simulink model "VACModel"  (Simulink 8.3)
settings: Solver=ode1  SolverMode=MultiTasking  StartTime=0.0  StopTime=24  FixedStep=Ts_base  MaxStep=Ts_base  MinStep=1e-6  RelTol=1e-6
PreLoadFcn:
  | initModel
StopFcn:
  | overview
undefined symbols (not defined in the file): automatic, controller_sampling_frequency, Fixed, gcr, MVs, PI, signal, transmitter_deadtime, transmitter_sampling_frequency, Ts_save, y_ss
libraries: VAlib x96
(part 12 of 18)

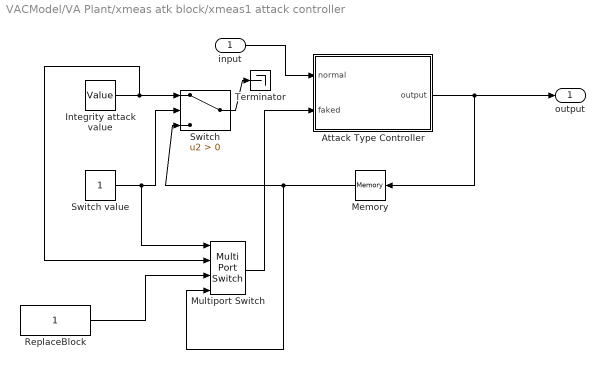
== system VACModel/VA Plant/xmeas atk block/xmeas1 attack controller ==
  input : Inport
  Attack Type Controller : Subsystem  Variant=on  OverrideUsingVariant=normal_forward_controller  mask{atkMode=No attack, start=0, duration=duration}
      mask prompts: atkMode "Attack Mode:"
      mask TypeOptions atkMode: No attack | Step attack | Interval attack | Periodical attack
      mask Callback atkMode:
      | switch get_param(gcb,'atkMode');
      |     case 'Step attack'
      |         set_param(gcb, 'OverrideUsingVariant', 'step_forward_controller');
      |     case 'Interval attack'
      |         set_param(gcb, 'OverrideUsingVariant', 'interval_forward_controller');
      |     case 'Periodical attack'
      |         set_param(gcb, 'OverrideUsingVariant', 'periodical_forward_controller');
      |     otherwise
      |         set_param(gcb, 'OverrideUsingVariant', 'normal_forward_controller');
      | end
      mask Display: eval(get_param([gcb '/' strrep(get_param(gcb, 'ActiveVariant'), '_', ' ')], 'MaskDisplay'));
  Integrity attack value : Constant  Value=Value
  Memory : Memory
  Multiport Switch : MultiPortSwitch
  ReplaceBlock : Constant
  Switch : Switch  Criteria=u2 > Threshold
  Switch value : Constant
  Terminator : Terminator
  output : Outport
  wires:
  ReplaceBlock/1 -> Multiport Switch/3
  Switch/1 -> Terminator/1
  Multiport Switch/1 -> Attack Type Controller/2(faked)
  Memory/1 -> Switch/3, Multiport Switch/4
  input/1 -> Attack Type Controller/1(normal)
  Switch value/1 -> Switch/2, Multiport Switch/1
  Attack Type Controller/1(output) -> output/1, Memory/1
  Integrity attack value/1 -> Switch/1, Multiport Switch/2

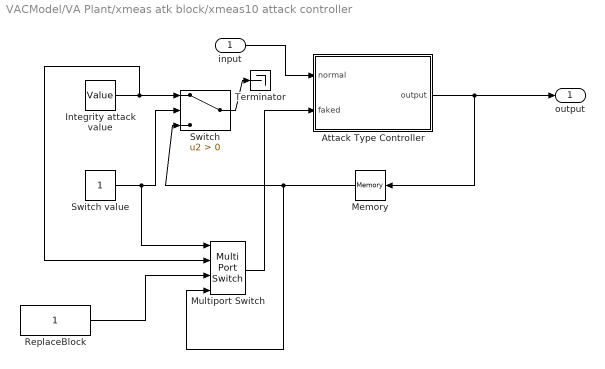
== system VACModel/VA Plant/xmeas atk block/xmeas10 attack controller ==
  input : Inport
  Attack Type Controller : Subsystem  Variant=on  OverrideUsingVariant=normal_forward_controller  mask{atkMode=No attack, start=0, duration=duration}
      mask prompts: atkMode "Attack Mode:"
      mask TypeOptions atkMode: No attack | Step attack | Interval attack | Periodical attack
      mask Callback atkMode:
      | switch get_param(gcb,'atkMode');
      |     case 'Step attack'
      |         set_param(gcb, 'OverrideUsingVariant', 'step_forward_controller');
      |     case 'Interval attack'
      |         set_param(gcb, 'OverrideUsingVariant', 'interval_forward_controller');
      |     case 'Periodical attack'
      |         set_param(gcb, 'OverrideUsingVariant', 'periodical_forward_controller');
      |     otherwise
      |         set_param(gcb, 'OverrideUsingVariant', 'normal_forward_controller');
      | end
      mask Display: eval(get_param([gcb '/' strrep(get_param(gcb, 'ActiveVariant'), '_', ' ')], 'MaskDisplay'));
  Integrity attack value : Constant  Value=Value
  Memory : Memory
  Multiport Switch : MultiPortSwitch
  ReplaceBlock : Constant
  Switch : Switch  Criteria=u2 > Threshold
  Switch value : Constant
  Terminator : Terminator
  output : Outport
  wires:
  ReplaceBlock/1 -> Multiport Switch/3
  Switch/1 -> Terminator/1
  Multiport Switch/1 -> Attack Type Controller/2(faked)
  Memory/1 -> Switch/3, Multiport Switch/4
  input/1 -> Attack Type Controller/1(normal)
  Switch value/1 -> Switch/2, Multiport Switch/1
  Attack Type Controller/1(output) -> output/1, Memory/1
  Integrity attack value/1 -> Switch/1, Multiport Switch/2

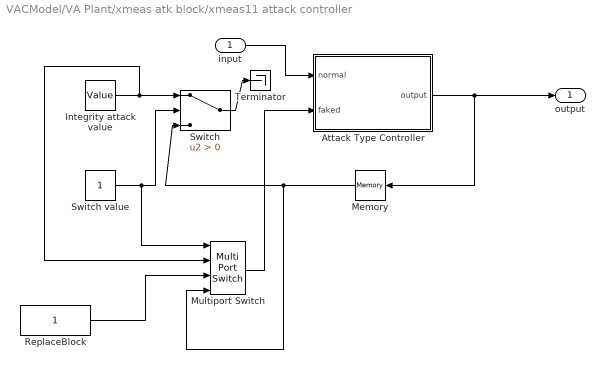
== system VACModel/VA Plant/xmeas atk block/xmeas11 attack controller ==
  input : Inport
  Attack Type Controller : Subsystem  Variant=on  OverrideUsingVariant=normal_forward_controller  mask{atkMode=No attack, start=0, duration=duration}
      mask prompts: atkMode "Attack Mode:"
      mask TypeOptions atkMode: No attack | Step attack | Interval attack | Periodical attack
      mask Callback atkMode:
      | switch get_param(gcb,'atkMode');
      |     case 'Step attack'
      |         set_param(gcb, 'OverrideUsingVariant', 'step_forward_controller');
      |     case 'Interval attack'
      |         set_param(gcb, 'OverrideUsingVariant', 'interval_forward_controller');
      |     case 'Periodical attack'
      |         set_param(gcb, 'OverrideUsingVariant', 'periodical_forward_controller');
      |     otherwise
      |         set_param(gcb, 'OverrideUsingVariant', 'normal_forward_controller');
      | end
      mask Display: eval(get_param([gcb '/' strrep(get_param(gcb, 'ActiveVariant'), '_', ' ')], 'MaskDisplay'));
  Integrity attack value : Constant  Value=Value
  Memory : Memory
  Multiport Switch : MultiPortSwitch
  ReplaceBlock : Constant
  Switch : Switch  Criteria=u2 > Threshold
  Switch value : Constant
  Terminator : Terminator
  output : Outport
  wires:
  ReplaceBlock/1 -> Multiport Switch/3
  Switch/1 -> Terminator/1
  Multiport Switch/1 -> Attack Type Controller/2(faked)
  Memory/1 -> Switch/3, Multiport Switch/4
  input/1 -> Attack Type Controller/1(normal)
  Switch value/1 -> Switch/2, Multiport Switch/1
  Attack Type Controller/1(output) -> output/1, Memory/1
  Integrity attack value/1 -> Switch/1, Multiport Switch/2

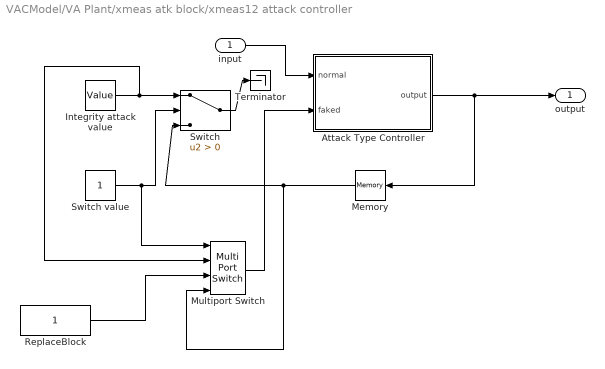
== system VACModel/VA Plant/xmeas atk block/xmeas12 attack controller ==
  input : Inport
  Attack Type Controller : Subsystem  Variant=on  OverrideUsingVariant=normal_forward_controller  mask{atkMode=No attack, start=0, duration=duration}
      mask prompts: atkMode "Attack Mode:"
      mask TypeOptions atkMode: No attack | Step attack | Interval attack | Periodical attack
      mask Callback atkMode:
      | switch get_param(gcb,'atkMode');
      |     case 'Step attack'
      |         set_param(gcb, 'OverrideUsingVariant', 'step_forward_controller');
      |     case 'Interval attack'
      |         set_param(gcb, 'OverrideUsingVariant', 'interval_forward_controller');
      |     case 'Periodical attack'
      |         set_param(gcb, 'OverrideUsingVariant', 'periodical_forward_controller');
      |     otherwise
      |         set_param(gcb, 'OverrideUsingVariant', 'normal_forward_controller');
      | end
      mask Display: eval(get_param([gcb '/' strrep(get_param(gcb, 'ActiveVariant'), '_', ' ')], 'MaskDisplay'));
  Integrity attack value : Constant  Value=Value
  Memory : Memory
  Multiport Switch : MultiPortSwitch
  ReplaceBlock : Constant
  Switch : Switch  Criteria=u2 > Threshold
  Switch value : Constant
  Terminator : Terminator
  output : Outport
  wires:
  ReplaceBlock/1 -> Multiport Switch/3
  Switch/1 -> Terminator/1
  Multiport Switch/1 -> Attack Type Controller/2(faked)
  Memory/1 -> Switch/3, Multiport Switch/4
  input/1 -> Attack Type Controller/1(normal)
  Switch value/1 -> Switch/2, Multiport Switch/1
  Attack Type Controller/1(output) -> output/1, Memory/1
  Integrity attack value/1 -> Switch/1, Multiport Switch/2

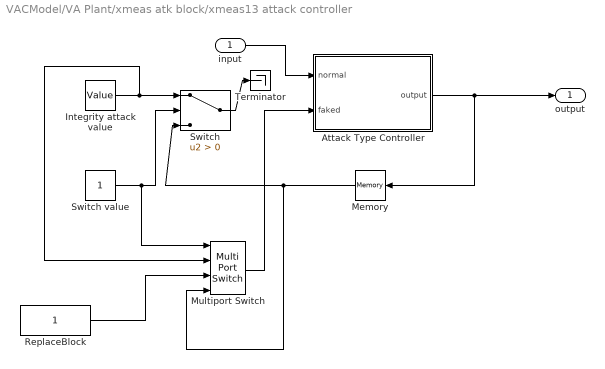
== system VACModel/VA Plant/xmeas atk block/xmeas13 attack controller ==
  input : Inport
  Attack Type Controller : Subsystem  Variant=on  OverrideUsingVariant=normal_forward_controller  mask{atkMode=No attack, start=0, duration=duration}
      mask prompts: atkMode "Attack Mode:"
      mask TypeOptions atkMode: No attack | Step attack | Interval attack | Periodical attack
      mask Callback atkMode:
      | switch get_param(gcb,'atkMode');
      |     case 'Step attack'
      |         set_param(gcb, 'OverrideUsingVariant', 'step_forward_controller');
      |     case 'Interval attack'
      |         set_param(gcb, 'OverrideUsingVariant', 'interval_forward_controller');
      |     case 'Periodical attack'
      |         set_param(gcb, 'OverrideUsingVariant', 'periodical_forward_controller');
      |     otherwise
      |         set_param(gcb, 'OverrideUsingVariant', 'normal_forward_controller');
      | end
      mask Display: eval(get_param([gcb '/' strrep(get_param(gcb, 'ActiveVariant'), '_', ' ')], 'MaskDisplay'));
  Integrity attack value : Constant  Value=Value
  Memory : Memory
  Multiport Switch : MultiPortSwitch
  ReplaceBlock : Constant
  Switch : Switch  Criteria=u2 > Threshold
  Switch value : Constant
  Terminator : Terminator
  output : Outport
  wires:
  ReplaceBlock/1 -> Multiport Switch/3
  Switch/1 -> Terminator/1
  Multiport Switch/1 -> Attack Type Controller/2(faked)
  Memory/1 -> Switch/3, Multiport Switch/4
  input/1 -> Attack Type Controller/1(normal)
  Switch value/1 -> Switch/2, Multiport Switch/1
  Attack Type Controller/1(output) -> output/1, Memory/1
  Integrity attack value/1 -> Switch/1, Multiport Switch/2

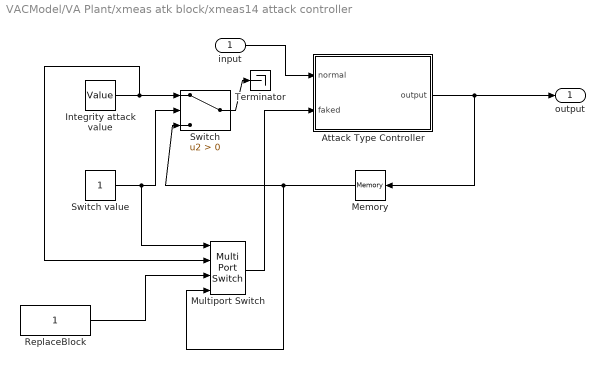
== system VACModel/VA Plant/xmeas atk block/xmeas14 attack controller ==
  input : Inport
  Attack Type Controller : Subsystem  Variant=on  OverrideUsingVariant=normal_forward_controller  mask{atkMode=No attack, start=0, duration=duration}
      mask prompts: atkMode "Attack Mode:"
      mask TypeOptions atkMode: No attack | Step attack | Interval attack | Periodical attack
      mask Callback atkMode:
      | switch get_param(gcb,'atkMode');
      |     case 'Step attack'
      |         set_param(gcb, 'OverrideUsingVariant', 'step_forward_controller');
      |     case 'Interval attack'
      |         set_param(gcb, 'OverrideUsingVariant', 'interval_forward_controller');
      |     case 'Periodical attack'
      |         set_param(gcb, 'OverrideUsingVariant', 'periodical_forward_controller');
      |     otherwise
      |         set_param(gcb, 'OverrideUsingVariant', 'normal_forward_controller');
      | end
      mask Display: eval(get_param([gcb '/' strrep(get_param(gcb, 'ActiveVariant'), '_', ' ')], 'MaskDisplay'));
  Integrity attack value : Constant  Value=Value
  Memory : Memory
  Multiport Switch : MultiPortSwitch
  ReplaceBlock : Constant
  Switch : Switch  Criteria=u2 > Threshold
  Switch value : Constant
  Terminator : Terminator
  output : Outport
  wires:
  ReplaceBlock/1 -> Multiport Switch/3
  Switch/1 -> Terminator/1
  Multiport Switch/1 -> Attack Type Controller/2(faked)
  Memory/1 -> Switch/3, Multiport Switch/4
  input/1 -> Attack Type Controller/1(normal)
  Switch value/1 -> Switch/2, Multiport Switch/1
  Attack Type Controller/1(output) -> output/1, Memory/1
  Integrity attack value/1 -> Switch/1, Multiport Switch/2

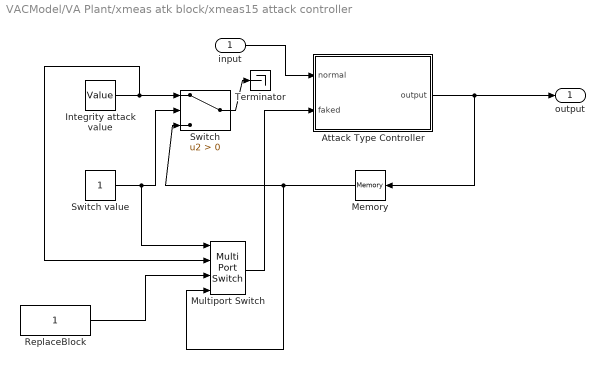
== system VACModel/VA Plant/xmeas atk block/xmeas15 attack controller ==
  input : Inport
  Attack Type Controller : Subsystem  Variant=on  OverrideUsingVariant=normal_forward_controller  mask{atkMode=No attack, start=0, duration=duration}
      mask prompts: atkMode "Attack Mode:"
      mask TypeOptions atkMode: No attack | Step attack | Interval attack | Periodical attack
      mask Callback atkMode:
      | switch get_param(gcb,'atkMode');
      |     case 'Step attack'
      |         set_param(gcb, 'OverrideUsingVariant', 'step_forward_controller');
      |     case 'Interval attack'
      |         set_param(gcb, 'OverrideUsingVariant', 'interval_forward_controller');
      |     case 'Periodical attack'
      |         set_param(gcb, 'OverrideUsingVariant', 'periodical_forward_controller');
      |     otherwise
      |         set_param(gcb, 'OverrideUsingVariant', 'normal_forward_controller');
      | end
      mask Display: eval(get_param([gcb '/' strrep(get_param(gcb, 'ActiveVariant'), '_', ' ')], 'MaskDisplay'));
  Integrity attack value : Constant  Value=Value
  Memory : Memory
  Multiport Switch : MultiPortSwitch
  ReplaceBlock : Constant
  Switch : Switch  Criteria=u2 > Threshold
  Switch value : Constant
  Terminator : Terminator
  output : Outport
  wires:
  ReplaceBlock/1 -> Multiport Switch/3
  Switch/1 -> Terminator/1
  Multiport Switch/1 -> Attack Type Controller/2(faked)
  Memory/1 -> Switch/3, Multiport Switch/4
  input/1 -> Attack Type Controller/1(normal)
  Switch value/1 -> Switch/2, Multiport Switch/1
  Attack Type Controller/1(output) -> output/1, Memory/1
  Integrity attack value/1 -> Switch/1, Multiport Switch/2

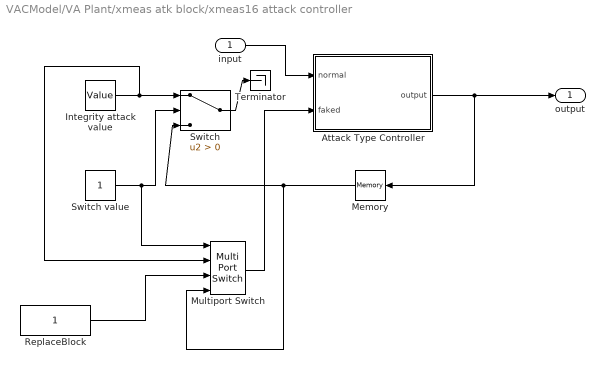
== system VACModel/VA Plant/xmeas atk block/xmeas16 attack controller ==
  input : Inport
  Attack Type Controller : Subsystem  Variant=on  OverrideUsingVariant=normal_forward_controller  mask{atkMode=No attack, start=0, duration=duration}
      mask prompts: atkMode "Attack Mode:"
      mask TypeOptions atkMode: No attack | Step attack | Interval attack | Periodical attack
      mask Callback atkMode:
      | switch get_param(gcb,'atkMode');
      |     case 'Step attack'
      |         set_param(gcb, 'OverrideUsingVariant', 'step_forward_controller');
      |     case 'Interval attack'
      |         set_param(gcb, 'OverrideUsingVariant', 'interval_forward_controller');
      |     case 'Periodical attack'
      |         set_param(gcb, 'OverrideUsingVariant', 'periodical_forward_controller');
      |     otherwise
      |         set_param(gcb, 'OverrideUsingVariant', 'normal_forward_controller');
      | end
      mask Display: eval(get_param([gcb '/' strrep(get_param(gcb, 'ActiveVariant'), '_', ' ')], 'MaskDisplay'));
  Integrity attack value : Constant  Value=Value
  Memory : Memory
  Multiport Switch : MultiPortSwitch
  ReplaceBlock : Constant
  Switch : Switch  Criteria=u2 > Threshold
  Switch value : Constant
  Terminator : Terminator
  output : Outport
  wires:
  ReplaceBlock/1 -> Multiport Switch/3
  Switch/1 -> Terminator/1
  Multiport Switch/1 -> Attack Type Controller/2(faked)
  Memory/1 -> Switch/3, Multiport Switch/4
  input/1 -> Attack Type Controller/1(normal)
  Switch value/1 -> Switch/2, Multiport Switch/1
  Attack Type Controller/1(output) -> output/1, Memory/1
  Integrity attack value/1 -> Switch/1, Multiport Switch/2

== system VACModel/VA Plant/xmeas atk block/xmeas17 attack controller ==
  input : Inport
  Attack Type Controller : Subsystem  Variant=on  OverrideUsingVariant=normal_forward_controller  mask{atkMode=No attack, start=0, duration=duration}
      mask prompts: atkMode "Attack Mode:"
      mask TypeOptions atkMode: No attack | Step attack | Interval attack | Periodical attack
      mask Callback atkMode:
      | switch get_param(gcb,'atkMode');
      |     case 'Step attack'
      |         set_param(gcb, 'OverrideUsingVariant', 'step_forward_controller');
      |     case 'Interval attack'
      |         set_param(gcb, 'OverrideUsingVariant', 'interval_forward_controller');
      |     case 'Periodical attack'
      |         set_param(gcb, 'OverrideUsingVariant', 'periodical_forward_controller');
      |     otherwise
      |         set_param(gcb, 'OverrideUsingVariant', 'normal_forward_controller');
      | end
      mask Display: eval(get_param([gcb '/' strrep(get_param(gcb, 'ActiveVariant'), '_', ' ')], 'MaskDisplay'));
  Integrity attack value : Constant  Value=Value
  Memory : Memory
  Multiport Switch : MultiPortSwitch
  ReplaceBlock : Constant
  Switch : Switch  Criteria=u2 > Threshold
  Switch value : Constant
  Terminator : Terminator
  output : Outport
  wires:
  ReplaceBlock/1 -> Multiport Switch/3
  Switch/1 -> Terminator/1
  Multiport Switch/1 -> Attack Type Controller/2(faked)
  Memory/1 -> Switch/3, Multiport Switch/4
  input/1 -> Attack Type Controller/1(normal)
  Switch value/1 -> Switch/2, Multiport Switch/1
  Attack Type Controller/1(output) -> output/1, Memory/1
  Integrity attack value/1 -> Switch/1, Multiport Switch/2

== system VACModel/VA Plant/xmeas atk block/xmeas18 attack controller ==
  input : Inport
  Attack Type Controller : Subsystem  Variant=on  OverrideUsingVariant=normal_forward_controller  mask{atkMode=No attack, start=0, duration=duration}
      mask prompts: atkMode "Attack Mode:"
      mask TypeOptions atkMode: No attack | Step attack | Interval attack | Periodical attack
      mask Callback atkMode:
      | switch get_param(gcb,'atkMode');
      |     case 'Step attack'
      |         set_param(gcb, 'OverrideUsingVariant', 'step_forward_controller');
      |     case 'Interval attack'
      |         set_param(gcb, 'OverrideUsingVariant', 'interval_forward_controller');
      |     case 'Periodical attack'
      |         set_param(gcb, 'OverrideUsingVariant', 'periodical_forward_controller');
      |     otherwise
      |         set_param(gcb, 'OverrideUsingVariant', 'normal_forward_controller');
      | end
      mask Display: eval(get_param([gcb '/' strrep(get_param(gcb, 'ActiveVariant'), '_', ' ')], 'MaskDisplay'));
  Integrity attack value : Constant  Value=Value
  Memory : Memory
  Multiport Switch : MultiPortSwitch
  ReplaceBlock : Constant
  Switch : Switch  Criteria=u2 > Threshold
  Switch value : Constant
  Terminator : Terminator
  output : Outport
  wires:
  ReplaceBlock/1 -> Multiport Switch/3
  Switch/1 -> Terminator/1
  Multiport Switch/1 -> Attack Type Controller/2(faked)
  Memory/1 -> Switch/3, Multiport Switch/4
  input/1 -> Attack Type Controller/1(normal)
  Switch value/1 -> Switch/2, Multiport Switch/1
  Attack Type Controller/1(output) -> output/1, Memory/1
  Integrity attack value/1 -> Switch/1, Multiport Switch/2

== system VACModel/VA Plant/xmeas atk block/xmeas19 attack controller ==
  input : Inport
  Attack Type Controller : Subsystem  Variant=on  OverrideUsingVariant=normal_forward_controller  mask{atkMode=No attack, start=0, duration=duration}
      mask prompts: atkMode "Attack Mode:"
      mask TypeOptions atkMode: No attack | Step attack | Interval attack | Periodical attack
      mask Callback atkMode:
      | switch get_param(gcb,'atkMode');
      |     case 'Step attack'
      |         set_param(gcb, 'OverrideUsingVariant', 'step_forward_controller');
      |     case 'Interval attack'
      |         set_param(gcb, 'OverrideUsingVariant', 'interval_forward_controller');
      |     case 'Periodical attack'
      |         set_param(gcb, 'OverrideUsingVariant', 'periodical_forward_controller');
      |     otherwise
      |         set_param(gcb, 'OverrideUsingVariant', 'normal_forward_controller');
      | end
      mask Display: eval(get_param([gcb '/' strrep(get_param(gcb, 'ActiveVariant'), '_', ' ')], 'MaskDisplay'));
  Integrity attack value : Constant  Value=Value
  Memory : Memory
  Multiport Switch : MultiPortSwitch
  ReplaceBlock : Constant
  Switch : Switch  Criteria=u2 > Threshold
  Switch value : Constant
  Terminator : Terminator
  output : Outport
  wires:
  ReplaceBlock/1 -> Multiport Switch/3
  Switch/1 -> Terminator/1
  Multiport Switch/1 -> Attack Type Controller/2(faked)
  Memory/1 -> Switch/3, Multiport Switch/4
  input/1 -> Attack Type Controller/1(normal)
  Switch value/1 -> Switch/2, Multiport Switch/1
  Attack Type Controller/1(output) -> output/1, Memory/1
  Integrity attack value/1 -> Switch/1, Multiport Switch/2

== system VACModel/VA Plant/xmeas atk block/xmeas2 attack controller ==
  input : Inport
  Attack Type Controller : Subsystem  Variant=on  OverrideUsingVariant=normal_forward_controller  mask{atkMode=No attack, start=0, duration=duration}
      mask prompts: atkMode "Attack Mode:"
      mask TypeOptions atkMode: No attack | Step attack | Interval attack | Periodical attack
      mask Callback atkMode:
      | switch get_param(gcb,'atkMode');
      |     case 'Step attack'
      |         set_param(gcb, 'OverrideUsingVariant', 'step_forward_controller');
      |     case 'Interval attack'
      |         set_param(gcb, 'OverrideUsingVariant', 'interval_forward_controller');
      |     case 'Periodical attack'
      |         set_param(gcb, 'OverrideUsingVariant', 'periodical_forward_controller');
      |     otherwise
      |         set_param(gcb, 'OverrideUsingVariant', 'normal_forward_controller');
      | end
      mask Display: eval(get_param([gcb '/' strrep(get_param(gcb, 'ActiveVariant'), '_', ' ')], 'MaskDisplay'));
  Integrity attack value : Constant  Value=Value
  Memory : Memory
  Multiport Switch : MultiPortSwitch
  ReplaceBlock : Constant
  Switch : Switch  Criteria=u2 > Threshold
  Switch value : Constant
  Terminator : Terminator
  output : Outport
  wires:
  ReplaceBlock/1 -> Multiport Switch/3
  Switch/1 -> Terminator/1
  Multiport Switch/1 -> Attack Type Controller/2(faked)
  Memory/1 -> Switch/3, Multiport Switch/4
  input/1 -> Attack Type Controller/1(normal)
  Switch value/1 -> Switch/2, Multiport Switch/1
  Attack Type Controller/1(output) -> output/1, Memory/1
  Integrity attack value/1 -> Switch/1, Multiport Switch/2

== system VACModel/VA Plant/xmeas atk block/xmeas20 attack controller ==
  input : Inport
  Attack Type Controller : Subsystem  Variant=on  OverrideUsingVariant=normal_forward_controller  mask{atkMode=No attack, start=0, duration=duration}
      mask prompts: atkMode "Attack Mode:"
      mask TypeOptions atkMode: No attack | Step attack | Interval attack | Periodical attack
      mask Callback atkMode:
      | switch get_param(gcb,'atkMode');
      |     case 'Step attack'
      |         set_param(gcb, 'OverrideUsingVariant', 'step_forward_controller');
      |     case 'Interval attack'
      |         set_param(gcb, 'OverrideUsingVariant', 'interval_forward_controller');
      |     case 'Periodical attack'
      |         set_param(gcb, 'OverrideUsingVariant', 'periodical_forward_controller');
      |     otherwise
      |         set_param(gcb, 'OverrideUsingVariant', 'normal_forward_controller');
      | end
      mask Display: eval(get_param([gcb '/' strrep(get_param(gcb, 'ActiveVariant'), '_', ' ')], 'MaskDisplay'));
  Integrity attack value : Constant  Value=Value
  Memory : Memory
  Multiport Switch : MultiPortSwitch
  ReplaceBlock : Constant
  Switch : Switch  Criteria=u2 > Threshold
  Switch value : Constant
  Terminator : Terminator
  output : Outport
  wires:
  ReplaceBlock/1 -> Multiport Switch/3
  Switch/1 -> Terminator/1
  Multiport Switch/1 -> Attack Type Controller/2(faked)
  Memory/1 -> Switch/3, Multiport Switch/4
  input/1 -> Attack Type Controller/1(normal)
  Switch value/1 -> Switch/2, Multiport Switch/1
  Attack Type Controller/1(output) -> output/1, Memory/1
  Integrity attack value/1 -> Switch/1, Multiport Switch/2

== system VACModel/VA Plant/xmeas atk block/xmeas21 attack controller ==
  input : Inport
  Attack Type Controller : Subsystem  Variant=on  OverrideUsingVariant=normal_forward_controller  mask{atkMode=No attack, start=0, duration=duration}
      mask prompts: atkMode "Attack Mode:"
      mask TypeOptions atkMode: No attack | Step attack | Interval attack | Periodical attack
      mask Callback atkMode:
      | switch get_param(gcb,'atkMode');
      |     case 'Step attack'
      |         set_param(gcb, 'OverrideUsingVariant', 'step_forward_controller');
      |     case 'Interval attack'
      |         set_param(gcb, 'OverrideUsingVariant', 'interval_forward_controller');
      |     case 'Periodical attack'
      |         set_param(gcb, 'OverrideUsingVariant', 'periodical_forward_controller');
      |     otherwise
      |         set_param(gcb, 'OverrideUsingVariant', 'normal_forward_controller');
      | end
      mask Display: eval(get_param([gcb '/' strrep(get_param(gcb, 'ActiveVariant'), '_', ' ')], 'MaskDisplay'));
  Integrity attack value : Constant  Value=Value
  Memory : Memory
  Multiport Switch : MultiPortSwitch
  ReplaceBlock : Constant
  Switch : Switch  Criteria=u2 > Threshold
  Switch value : Constant
  Terminator : Terminator
  output : Outport
  wires:
  ReplaceBlock/1 -> Multiport Switch/3
  Switch/1 -> Terminator/1
  Multiport Switch/1 -> Attack Type Controller/2(faked)
  Memory/1 -> Switch/3, Multiport Switch/4
  input/1 -> Attack Type Controller/1(normal)
  Switch value/1 -> Switch/2, Multiport Switch/1
  Attack Type Controller/1(output) -> output/1, Memory/1
  Integrity attack value/1 -> Switch/1, Multiport Switch/2

== system VACModel/VA Plant/xmeas atk block/xmeas22 attack controller ==
  input : Inport
  Attack Type Controller : Subsystem  Variant=on  OverrideUsingVariant=normal_forward_controller  mask{atkMode=No attack, start=0, duration=duration}
      mask prompts: atkMode "Attack Mode:"
      mask TypeOptions atkMode: No attack | Step attack | Interval attack | Periodical attack
      mask Callback atkMode:
      | switch get_param(gcb,'atkMode');
      |     case 'Step attack'
      |         set_param(gcb, 'OverrideUsingVariant', 'step_forward_controller');
      |     case 'Interval attack'
      |         set_param(gcb, 'OverrideUsingVariant', 'interval_forward_controller');
      |     case 'Periodical attack'
      |         set_param(gcb, 'OverrideUsingVariant', 'periodical_forward_controller');
      |     otherwise
      |         set_param(gcb, 'OverrideUsingVariant', 'normal_forward_controller');
      | end
      mask Display: eval(get_param([gcb '/' strrep(get_param(gcb, 'ActiveVariant'), '_', ' ')], 'MaskDisplay'));
  Integrity attack value : Constant  Value=Value
  Memory : Memory
  Multiport Switch : MultiPortSwitch
  ReplaceBlock : Constant
  Switch : Switch  Criteria=u2 > Threshold
  Switch value : Constant
  Terminator : Terminator
  output : Outport
  wires:
  ReplaceBlock/1 -> Multiport Switch/3
  Switch/1 -> Terminator/1
  Multiport Switch/1 -> Attack Type Controller/2(faked)
  Memory/1 -> Switch/3, Multiport Switch/4
  input/1 -> Attack Type Controller/1(normal)
  Switch value/1 -> Switch/2, Multiport Switch/1
  Attack Type Controller/1(output) -> output/1, Memory/1
  Integrity attack value/1 -> Switch/1, Multiport Switch/2

== system VACModel/VA Plant/xmeas atk block/xmeas23 attack controller ==
  input : Inport
  Attack Type Controller : Subsystem  Variant=on  OverrideUsingVariant=normal_forward_controller  mask{atkMode=No attack, start=0, duration=duration}
      mask prompts: atkMode "Attack Mode:"
      mask TypeOptions atkMode: No attack | Step attack | Interval attack | Periodical attack
      mask Callback atkMode:
      | switch get_param(gcb,'atkMode');
      |     case 'Step attack'
      |         set_param(gcb, 'OverrideUsingVariant', 'step_forward_controller');
      |     case 'Interval attack'
      |         set_param(gcb, 'OverrideUsingVariant', 'interval_forward_controller');
      |     case 'Periodical attack'
      |         set_param(gcb, 'OverrideUsingVariant', 'periodical_forward_controller');
      |     otherwise
      |         set_param(gcb, 'OverrideUsingVariant', 'normal_forward_controller');
      | end
      mask Display: eval(get_param([gcb '/' strrep(get_param(gcb, 'ActiveVariant'), '_', ' ')], 'MaskDisplay'));
  Integrity attack value : Constant  Value=Value
  Memory : Memory
  Multiport Switch : MultiPortSwitch
  ReplaceBlock : Constant
  Switch : Switch  Criteria=u2 > Threshold
  Switch value : Constant
  Terminator : Terminator
  output : Outport
  wires:
  ReplaceBlock/1 -> Multiport Switch/3
  Switch/1 -> Terminator/1
  Multiport Switch/1 -> Attack Type Controller/2(faked)
  Memory/1 -> Switch/3, Multiport Switch/4
  input/1 -> Attack Type Controller/1(normal)
  Switch value/1 -> Switch/2, Multiport Switch/1
  Attack Type Controller/1(output) -> output/1, Memory/1
  Integrity attack value/1 -> Switch/1, Multiport Switch/2

== system VACModel/VA Plant/xmeas atk block/xmeas24 attack controller ==
  input : Inport
  Attack Type Controller : Subsystem  Variant=on  OverrideUsingVariant=normal_forward_controller  mask{atkMode=No attack, start=0, duration=duration}
      mask prompts: atkMode "Attack Mode:"
      mask TypeOptions atkMode: No attack | Step attack | Interval attack | Periodical attack
      mask Callback atkMode:
      | switch get_param(gcb,'atkMode');
      |     case 'Step attack'
      |         set_param(gcb, 'OverrideUsingVariant', 'step_forward_controller');
      |     case 'Interval attack'
      |         set_param(gcb, 'OverrideUsingVariant', 'interval_forward_controller');
      |     case 'Periodical attack'
      |         set_param(gcb, 'OverrideUsingVariant', 'periodical_forward_controller');
      |     otherwise
      |         set_param(gcb, 'OverrideUsingVariant', 'normal_forward_controller');
      | end
      mask Display: eval(get_param([gcb '/' strrep(get_param(gcb, 'ActiveVariant'), '_', ' ')], 'MaskDisplay'));
  Integrity attack value : Constant  Value=Value
  Memory : Memory
  Multiport Switch : MultiPortSwitch
  ReplaceBlock : Constant
  Switch : Switch  Criteria=u2 > Threshold
  Switch value : Constant
  Terminator : Terminator
  output : Outport
  wires:
  ReplaceBlock/1 -> Multiport Switch/3
  Switch/1 -> Terminator/1
  Multiport Switch/1 -> Attack Type Controller/2(faked)
  Memory/1 -> Switch/3, Multiport Switch/4
  input/1 -> Attack Type Controller/1(normal)
  Switch value/1 -> Switch/2, Multiport Switch/1
  Attack Type Controller/1(output) -> output/1, Memory/1
  Integrity attack value/1 -> Switch/1, Multiport Switch/2

== system VACModel/VA Plant/xmeas atk block/xmeas25 attack controller ==
  input : Inport
  Attack Type Controller : Subsystem  Variant=on  OverrideUsingVariant=normal_forward_controller  mask{atkMode=No attack, start=0, duration=duration}
      mask prompts: atkMode "Attack Mode:"
      mask TypeOptions atkMode: No attack | Step attack | Interval attack | Periodical attack
      mask Callback atkMode:
      | switch get_param(gcb,'atkMode');
      |     case 'Step attack'
      |         set_param(gcb, 'OverrideUsingVariant', 'step_forward_controller');
      |     case 'Interval attack'
      |         set_param(gcb, 'OverrideUsingVariant', 'interval_forward_controller');
      |     case 'Periodical attack'
      |         set_param(gcb, 'OverrideUsingVariant', 'periodical_forward_controller');
      |     otherwise
      |         set_param(gcb, 'OverrideUsingVariant', 'normal_forward_controller');
      | end
      mask Display: eval(get_param([gcb '/' strrep(get_param(gcb, 'ActiveVariant'), '_', ' ')], 'MaskDisplay'));
  Integrity attack value : Constant  Value=Value
  Memory : Memory
  Multiport Switch : MultiPortSwitch
  ReplaceBlock : Constant
  Switch : Switch  Criteria=u2 > Threshold
  Switch value : Constant
  Terminator : Terminator
  output : Outport
  wires:
  ReplaceBlock/1 -> Multiport Switch/3
  Switch/1 -> Terminator/1
  Multiport Switch/1 -> Attack Type Controller/2(faked)
  Memory/1 -> Switch/3, Multiport Switch/4
  input/1 -> Attack Type Controller/1(normal)
  Switch value/1 -> Switch/2, Multiport Switch/1
  Attack Type Controller/1(output) -> output/1, Memory/1
  Integrity attack value/1 -> Switch/1, Multiport Switch/2

== system VACModel/VA Plant/xmeas atk block/xmeas26 attack controller ==
  input : Inport
  Attack Type Controller : Subsystem  Variant=on  OverrideUsingVariant=normal_forward_controller  mask{atkMode=No attack, start=0, duration=duration}
      mask prompts: atkMode "Attack Mode:"
      mask TypeOptions atkMode: No attack | Step attack | Interval attack | Periodical attack
      mask Callback atkMode:
      | switch get_param(gcb,'atkMode');
      |     case 'Step attack'
      |         set_param(gcb, 'OverrideUsingVariant', 'step_forward_controller');
      |     case 'Interval attack'
      |         set_param(gcb, 'OverrideUsingVariant', 'interval_forward_controller');
      |     case 'Periodical attack'
      |         set_param(gcb, 'OverrideUsingVariant', 'periodical_forward_controller');
      |     otherwise
      |         set_param(gcb, 'OverrideUsingVariant', 'normal_forward_controller');
      | end
      mask Display: eval(get_param([gcb '/' strrep(get_param(gcb, 'ActiveVariant'), '_', ' ')], 'MaskDisplay'));
  Integrity attack value : Constant  Value=Value
  Memory : Memory
  Multiport Switch : MultiPortSwitch
  ReplaceBlock : Constant
  Switch : Switch  Criteria=u2 > Threshold
  Switch value : Constant
  Terminator : Terminator
  output : Outport
  wires:
  ReplaceBlock/1 -> Multiport Switch/3
  Switch/1 -> Terminator/1
  Multiport Switch/1 -> Attack Type Controller/2(faked)
  Memory/1 -> Switch/3, Multiport Switch/4
  input/1 -> Attack Type Controller/1(normal)
  Switch value/1 -> Switch/2, Multiport Switch/1
  Attack Type Controller/1(output) -> output/1, Memory/1
  Integrity attack value/1 -> Switch/1, Multiport Switch/2

== system VACModel/VA Plant/xmeas atk block/xmeas27 attack controller ==
  input : Inport
  Attack Type Controller : Subsystem  Variant=on  OverrideUsingVariant=normal_forward_controller  mask{atkMode=No attack, start=0, duration=duration}
      mask prompts: atkMode "Attack Mode:"
      mask TypeOptions atkMode: No attack | Step attack | Interval attack | Periodical attack
      mask Callback atkMode:
      | switch get_param(gcb,'atkMode');
      |     case 'Step attack'
      |         set_param(gcb, 'OverrideUsingVariant', 'step_forward_controller');
      |     case 'Interval attack'
      |         set_param(gcb, 'OverrideUsingVariant', 'interval_forward_controller');
      |     case 'Periodical attack'
      |         set_param(gcb, 'OverrideUsingVariant', 'periodical_forward_controller');
      |     otherwise
      |         set_param(gcb, 'OverrideUsingVariant', 'normal_forward_controller');
      | end
      mask Display: eval(get_param([gcb '/' strrep(get_param(gcb, 'ActiveVariant'), '_', ' ')], 'MaskDisplay'));
  Integrity attack value : Constant  Value=Value
  Memory : Memory
  Multiport Switch : MultiPortSwitch
  ReplaceBlock : Constant
  Switch : Switch  Criteria=u2 > Threshold
  Switch value : Constant
  Terminator : Terminator
  output : Outport
  wires:
  ReplaceBlock/1 -> Multiport Switch/3
  Switch/1 -> Terminator/1
  Multiport Switch/1 -> Attack Type Controller/2(faked)
  Memory/1 -> Switch/3, Multiport Switch/4
  input/1 -> Attack Type Controller/1(normal)
  Switch value/1 -> Switch/2, Multiport Switch/1
  Attack Type Controller/1(output) -> output/1, Memory/1
  Integrity attack value/1 -> Switch/1, Multiport Switch/2

== system VACModel/VA Plant/xmeas atk block/xmeas28 attack controller ==
  input : Inport
  Attack Type Controller : Subsystem  Variant=on  OverrideUsingVariant=normal_forward_controller  mask{atkMode=No attack, start=0, duration=duration}
      mask prompts: atkMode "Attack Mode:"
      mask TypeOptions atkMode: No attack | Step attack | Interval attack | Periodical attack
      mask Callback atkMode:
      | switch get_param(gcb,'atkMode');
      |     case 'Step attack'
      |         set_param(gcb, 'OverrideUsingVariant', 'step_forward_controller');
      |     case 'Interval attack'
      |         set_param(gcb, 'OverrideUsingVariant', 'interval_forward_controller');
      |     case 'Periodical attack'
      |         set_param(gcb, 'OverrideUsingVariant', 'periodical_forward_controller');
      |     otherwise
      |         set_param(gcb, 'OverrideUsingVariant', 'normal_forward_controller');
      | end
      mask Display: eval(get_param([gcb '/' strrep(get_param(gcb, 'ActiveVariant'), '_', ' ')], 'MaskDisplay'));
  Integrity attack value : Constant  Value=Value
  Memory : Memory
  Multiport Switch : MultiPortSwitch
  ReplaceBlock : Constant
  Switch : Switch  Criteria=u2 > Threshold
  Switch value : Constant
  Terminator : Terminator
  output : Outport
  wires:
  ReplaceBlock/1 -> Multiport Switch/3
  Switch/1 -> Terminator/1
  Multiport Switch/1 -> Attack Type Controller/2(faked)
  Memory/1 -> Switch/3, Multiport Switch/4
  input/1 -> Attack Type Controller/1(normal)
  Switch value/1 -> Switch/2, Multiport Switch/1
  Attack Type Controller/1(output) -> output/1, Memory/1
  Integrity attack value/1 -> Switch/1, Multiport Switch/2

== system VACModel/VA Plant/xmeas atk block/xmeas29 attack controller ==
  input : Inport
  Attack Type Controller : Subsystem  Variant=on  OverrideUsingVariant=normal_forward_controller  mask{atkMode=No attack, start=0, duration=duration}
      mask prompts: atkMode "Attack Mode:"
      mask TypeOptions atkMode: No attack | Step attack | Interval attack | Periodical attack
      mask Callback atkMode:
      | switch get_param(gcb,'atkMode');
      |     case 'Step attack'
      |         set_param(gcb, 'OverrideUsingVariant', 'step_forward_controller');
      |     case 'Interval attack'
      |         set_param(gcb, 'OverrideUsingVariant', 'interval_forward_controller');
      |     case 'Periodical attack'
      |         set_param(gcb, 'OverrideUsingVariant', 'periodical_forward_controller');
      |     otherwise
      |         set_param(gcb, 'OverrideUsingVariant', 'normal_forward_controller');
      | end
      mask Display: eval(get_param([gcb '/' strrep(get_param(gcb, 'ActiveVariant'), '_', ' ')], 'MaskDisplay'));
  Integrity attack value : Constant  Value=Value
  Memory : Memory
  Multiport Switch : MultiPortSwitch
  ReplaceBlock : Constant
  Switch : Switch  Criteria=u2 > Threshold
  Switch value : Constant
  Terminator : Terminator
  output : Outport
  wires:
  ReplaceBlock/1 -> Multiport Switch/3
  Switch/1 -> Terminator/1
  Multiport Switch/1 -> Attack Type Controller/2(faked)
  Memory/1 -> Switch/3, Multiport Switch/4
  input/1 -> Attack Type Controller/1(normal)
  Switch value/1 -> Switch/2, Multiport Switch/1
  Attack Type Controller/1(output) -> output/1, Memory/1
  Integrity attack value/1 -> Switch/1, Multiport Switch/2

== system VACModel/VA Plant/xmeas atk block/xmeas3 attack controller ==
  input : Inport
  Attack Type Controller : Subsystem  Variant=on  OverrideUsingVariant=normal_forward_controller  mask{atkMode=No attack, start=0, duration=duration}
      mask prompts: atkMode "Attack Mode:"
      mask TypeOptions atkMode: No attack | Step attack | Interval attack | Periodical attack
      mask Callback atkMode:
      | switch get_param(gcb,'atkMode');
      |     case 'Step attack'
      |         set_param(gcb, 'OverrideUsingVariant', 'step_forward_controller');
      |     case 'Interval attack'
      |         set_param(gcb, 'OverrideUsingVariant', 'interval_forward_controller');
      |     case 'Periodical attack'
      |         set_param(gcb, 'OverrideUsingVariant', 'periodical_forward_controller');
      |     otherwise
      |         set_param(gcb, 'OverrideUsingVariant', 'normal_forward_controller');
      | end
      mask Display: eval(get_param([gcb '/' strrep(get_param(gcb, 'ActiveVariant'), '_', ' ')], 'MaskDisplay'));
  Integrity attack value : Constant  Value=Value
  Memory : Memory
  Multiport Switch : MultiPortSwitch
  ReplaceBlock : Constant
  Switch : Switch  Criteria=u2 > Threshold
  Switch value : Constant
  Terminator : Terminator
  output : Outport
  wires:
  ReplaceBlock/1 -> Multiport Switch/3
  Switch/1 -> Terminator/1
  Multiport Switch/1 -> Attack Type Controller/2(faked)
  Memory/1 -> Switch/3, Multiport Switch/4
  input/1 -> Attack Type Controller/1(normal)
  Switch value/1 -> Switch/2, Multiport Switch/1
  Attack Type Controller/1(output) -> output/1, Memory/1
  Integrity attack value/1 -> Switch/1, Multiport Switch/2

== system VACModel/VA Plant/xmeas atk block/xmeas30 attack controller ==
  input : Inport
  Attack Type Controller : Subsystem  Variant=on  OverrideUsingVariant=normal_forward_controller  mask{atkMode=No attack, start=0, duration=duration}
      mask prompts: atkMode "Attack Mode:"
      mask TypeOptions atkMode: No attack | Step attack | Interval attack | Periodical attack
      mask Callback atkMode:
      | switch get_param(gcb,'atkMode');
      |     case 'Step attack'
      |         set_param(gcb, 'OverrideUsingVariant', 'step_forward_controller');
      |     case 'Interval attack'
      |         set_param(gcb, 'OverrideUsingVariant', 'interval_forward_controller');
      |     case 'Periodical attack'
      |         set_param(gcb, 'OverrideUsingVariant', 'periodical_forward_controller');
      |     otherwise
      |         set_param(gcb, 'OverrideUsingVariant', 'normal_forward_controller');
      | end
      mask Display: eval(get_param([gcb '/' strrep(get_param(gcb, 'ActiveVariant'), '_', ' ')], 'MaskDisplay'));
  Integrity attack value : Constant  Value=Value
  Memory : Memory
  Multiport Switch : MultiPortSwitch
  ReplaceBlock : Constant
  Switch : Switch  Criteria=u2 > Threshold
  Switch value : Constant
  Terminator : Terminator
  output : Outport
  wires:
  ReplaceBlock/1 -> Multiport Switch/3
  Switch/1 -> Terminator/1
  Multiport Switch/1 -> Attack Type Controller/2(faked)
  Memory/1 -> Switch/3, Multiport Switch/4
  input/1 -> Attack Type Controller/1(normal)
  Switch value/1 -> Switch/2, Multiport Switch/1
  Attack Type Controller/1(output) -> output/1, Memory/1
  Integrity attack value/1 -> Switch/1, Multiport Switch/2

== system VACModel/VA Plant/xmeas atk block/xmeas31 attack controller ==
  input : Inport
  Attack Type Controller : Subsystem  Variant=on  OverrideUsingVariant=normal_forward_controller  mask{atkMode=No attack, start=0, duration=duration}
      mask prompts: atkMode "Attack Mode:"
      mask TypeOptions atkMode: No attack | Step attack | Interval attack | Periodical attack
      mask Callback atkMode:
      | switch get_param(gcb,'atkMode');
      |     case 'Step attack'
      |         set_param(gcb, 'OverrideUsingVariant', 'step_forward_controller');
      |     case 'Interval attack'
      |         set_param(gcb, 'OverrideUsingVariant', 'interval_forward_controller');
      |     case 'Periodical attack'
      |         set_param(gcb, 'OverrideUsingVariant', 'periodical_forward_controller');
      |     otherwise
      |         set_param(gcb, 'OverrideUsingVariant', 'normal_forward_controller');
      | end
      mask Display: eval(get_param([gcb '/' strrep(get_param(gcb, 'ActiveVariant'), '_', ' ')], 'MaskDisplay'));
  Integrity attack value : Constant  Value=Value
  Memory : Memory
  Multiport Switch : MultiPortSwitch
  ReplaceBlock : Constant
  Switch : Switch  Criteria=u2 > Threshold
  Switch value : Constant
  Terminator : Terminator
  output : Outport
  wires:
  ReplaceBlock/1 -> Multiport Switch/3
  Switch/1 -> Terminator/1
  Multiport Switch/1 -> Attack Type Controller/2(faked)
  Memory/1 -> Switch/3, Multiport Switch/4
  input/1 -> Attack Type Controller/1(normal)
  Switch value/1 -> Switch/2, Multiport Switch/1
  Attack Type Controller/1(output) -> output/1, Memory/1
  Integrity attack value/1 -> Switch/1, Multiport Switch/2

== system VACModel/VA Plant/xmeas atk block/xmeas32 attack controller ==
  input : Inport
  Attack Type Controller : Subsystem  Variant=on  OverrideUsingVariant=normal_forward_controller  mask{atkMode=No attack, start=0, duration=duration}
      mask prompts: atkMode "Attack Mode:"
      mask TypeOptions atkMode: No attack | Step attack | Interval attack | Periodical attack
      mask Callback atkMode:
      | switch get_param(gcb,'atkMode');
      |     case 'Step attack'
      |         set_param(gcb, 'OverrideUsingVariant', 'step_forward_controller');
      |     case 'Interval attack'
      |         set_param(gcb, 'OverrideUsingVariant', 'interval_forward_controller');
      |     case 'Periodical attack'
      |         set_param(gcb, 'OverrideUsingVariant', 'periodical_forward_controller');
      |     otherwise
      |         set_param(gcb, 'OverrideUsingVariant', 'normal_forward_controller');
      | end
      mask Display: eval(get_param([gcb '/' strrep(get_param(gcb, 'ActiveVariant'), '_', ' ')], 'MaskDisplay'));
  Integrity attack value : Constant  Value=Value
  Memory : Memory
  Multiport Switch : MultiPortSwitch
  ReplaceBlock : Constant
  Switch : Switch  Criteria=u2 > Threshold
  Switch value : Constant
  Terminator : Terminator
  output : Outport
  wires:
  ReplaceBlock/1 -> Multiport Switch/3
  Switch/1 -> Terminator/1
  Multiport Switch/1 -> Attack Type Controller/2(faked)
  Memory/1 -> Switch/3, Multiport Switch/4
  input/1 -> Attack Type Controller/1(normal)
  Switch value/1 -> Switch/2, Multiport Switch/1
  Attack Type Controller/1(output) -> output/1, Memory/1
  Integrity attack value/1 -> Switch/1, Multiport Switch/2

== system VACModel/VA Plant/xmeas atk block/xmeas33 attack controller ==
  input : Inport
  Attack Type Controller : Subsystem  Variant=on  OverrideUsingVariant=normal_forward_controller  mask{atkMode=No attack, start=0, duration=duration}
      mask prompts: atkMode "Attack Mode:"
      mask TypeOptions atkMode: No attack | Step attack | Interval attack | Periodical attack
      mask Callback atkMode:
      | switch get_param(gcb,'atkMode');
      |     case 'Step attack'
      |         set_param(gcb, 'OverrideUsingVariant', 'step_forward_controller');
      |     case 'Interval attack'
      |         set_param(gcb, 'OverrideUsingVariant', 'interval_forward_controller');
      |     case 'Periodical attack'
      |         set_param(gcb, 'OverrideUsingVariant', 'periodical_forward_controller');
      |     otherwise
      |         set_param(gcb, 'OverrideUsingVariant', 'normal_forward_controller');
      | end
      mask Display: eval(get_param([gcb '/' strrep(get_param(gcb, 'ActiveVariant'), '_', ' ')], 'MaskDisplay'));
  Integrity attack value : Constant  Value=Value
  Memory : Memory
  Multiport Switch : MultiPortSwitch
  ReplaceBlock : Constant
  Switch : Switch  Criteria=u2 > Threshold
  Switch value : Constant
  Terminator : Terminator
  output : Outport
  wires:
  ReplaceBlock/1 -> Multiport Switch/3
  Switch/1 -> Terminator/1
  Multiport Switch/1 -> Attack Type Controller/2(faked)
  Memory/1 -> Switch/3, Multiport Switch/4
  input/1 -> Attack Type Controller/1(normal)
  Switch value/1 -> Switch/2, Multiport Switch/1
  Attack Type Controller/1(output) -> output/1, Memory/1
  Integrity attack value/1 -> Switch/1, Multiport Switch/2

== system VACModel/VA Plant/xmeas atk block/xmeas34 attack controller ==
  input : Inport
  Attack Type Controller : Subsystem  Variant=on  OverrideUsingVariant=normal_forward_controller  mask{atkMode=No attack, start=0, duration=duration}
      mask prompts: atkMode "Attack Mode:"
      mask TypeOptions atkMode: No attack | Step attack | Interval attack | Periodical attack
      mask Callback atkMode:
      | switch get_param(gcb,'atkMode');
      |     case 'Step attack'
      |         set_param(gcb, 'OverrideUsingVariant', 'step_forward_controller');
      |     case 'Interval attack'
      |         set_param(gcb, 'OverrideUsingVariant', 'interval_forward_controller');
      |     case 'Periodical attack'
      |         set_param(gcb, 'OverrideUsingVariant', 'periodical_forward_controller');
      |     otherwise
      |         set_param(gcb, 'OverrideUsingVariant', 'normal_forward_controller');
      | end
      mask Display: eval(get_param([gcb '/' strrep(get_param(gcb, 'ActiveVariant'), '_', ' ')], 'MaskDisplay'));
  Integrity attack value : Constant  Value=Value
  Memory : Memory
  Multiport Switch : MultiPortSwitch
  ReplaceBlock : Constant
  Switch : Switch  Criteria=u2 > Threshold
  Switch value : Constant
  Terminator : Terminator
  output : Outport
  wires:
  ReplaceBlock/1 -> Multiport Switch/3
  Switch/1 -> Terminator/1
  Multiport Switch/1 -> Attack Type Controller/2(faked)
  Memory/1 -> Switch/3, Multiport Switch/4
  input/1 -> Attack Type Controller/1(normal)
  Switch value/1 -> Switch/2, Multiport Switch/1
  Attack Type Controller/1(output) -> output/1, Memory/1
  Integrity attack value/1 -> Switch/1, Multiport Switch/2

== system VACModel/VA Plant/xmeas atk block/xmeas35 attack controller ==
  input : Inport
  Attack Type Controller : Subsystem  Variant=on  OverrideUsingVariant=normal_forward_controller  mask{atkMode=No attack, start=0, duration=duration}
      mask prompts: atkMode "Attack Mode:"
      mask TypeOptions atkMode: No attack | Step attack | Interval attack | Periodical attack
      mask Callback atkMode:
      | switch get_param(gcb,'atkMode');
      |     case 'Step attack'
      |         set_param(gcb, 'OverrideUsingVariant', 'step_forward_controller');
      |     case 'Interval attack'
      |         set_param(gcb, 'OverrideUsingVariant', 'interval_forward_controller');
      |     case 'Periodical attack'
      |         set_param(gcb, 'OverrideUsingVariant', 'periodical_forward_controller');
      |     otherwise
      |         set_param(gcb, 'OverrideUsingVariant', 'normal_forward_controller');
      | end
      mask Display: eval(get_param([gcb '/' strrep(get_param(gcb, 'ActiveVariant'), '_', ' ')], 'MaskDisplay'));
  Integrity attack value : Constant  Value=Value
  Memory : Memory
  Multiport Switch : MultiPortSwitch
  ReplaceBlock : Constant
  Switch : Switch  Criteria=u2 > Threshold
  Switch value : Constant
  Terminator : Terminator
  output : Outport
  wires:
  ReplaceBlock/1 -> Multiport Switch/3
  Switch/1 -> Terminator/1
  Multiport Switch/1 -> Attack Type Controller/2(faked)
  Memory/1 -> Switch/3, Multiport Switch/4
  input/1 -> Attack Type Controller/1(normal)
  Switch value/1 -> Switch/2, Multiport Switch/1
  Attack Type Controller/1(output) -> output/1, Memory/1
  Integrity attack value/1 -> Switch/1, Multiport Switch/2
